simulink model "modeFinalPP"  (R2021b)
settings: Solver=ode23s  StartTime=0.0  StopTime=150  RelTol=1e-3
model workspace (MAT data in the model file):
  firstWarning = 1
  originalScenarioChecksum = '114339432DE22364D47BB28FC96DC10C'
undefined symbols (not defined in the file or in its folder): Acceleration, ActorID, AngularVelocity, curvature, DefaultGear, DEND_B, DEND_S, DEND_T, direction, gradbp, L, ld, LF, LR, MAX_BRAKE, MAX_STEER, MAX_TORQUE, MCAR, MIN_BRAKE, MIN_STEER, MIN_TORQUE, NUMD_B, NUMD_S, NUMD_T, Pitch, point_intersection, PoseRef, Position, psi_o, R, Roll, RRdamp, scenario, sigbuilder_block, STEER_RATIO, stopSign_ID, Tdead, thetaRefs, TL_ID, TrackWidth, Ts, ts, Vdead, Velocity, X_o, xRef2s, Y_o, Yaw, yRef2s
libraries: drivingvehiclecontroller x2, simulink x2, drivingscenarioandsensors x2, simulink_extras x1, autolibshared x1, vehdynlibviscommon x1, vehdynlibsteering x1
(part 2 of 2)

== stateflow chart modeFinalPP/Chart ==
  state Navigation
    state RailCrossing
      state Approaching
        en,du:
        VelCmd = ApproachingSpeed;
      state Stop
        en,du:
        VelCmd = 0;
        % apply brakes directly?
      state ExitScene
        en,du:
        ExitFlag = 1;
      state Transition
        en,du:
        VelCmd = SceneSpeed;
      (default) -> Navigation.RailCrossing.Approaching
      Navigation.RailCrossing.Approaching -> Navigation.RailCrossing.Stop : [D2S <= SDist]
      Navigation.RailCrossing.Stop -> Navigation.RailCrossing.Transition : [after(3,sec)]
      Navigation.RailCrossing.Transition -> Navigation.RailCrossing.ExitScene : [SDir == 'S']
    state RoundAbout
      state Approaching
        en,du:
        VelCmd = ApproachingSpeed;
      state Stop
        en,du:
        VelCmd = 0;
        % apply brakes directly?
      state ExitScene
        en,du:
        ExitFlag = 1;
      state Transition
        en,du:
        VelCmd = SceneSpeed;
      (default) -> Navigation.RoundAbout.Approaching
      Navigation.RoundAbout.Approaching -> Navigation.RoundAbout.Stop : [D2S <= SDist]
      Navigation.RoundAbout.Stop -> Navigation.RoundAbout.Transition : [after(3,sec)]
      Navigation.RoundAbout.Transition -> Navigation.RoundAbout.ExitScene : [SDir == 'S']
    state DestCheck
      en,du:
      % dest reached?
      (default) -> (junction 47)
      (junction 47) -> (junction 48) [order 1] : [D2D < 1]
      (junction 47) -> (junction 49) [order 2] : {DestReached = 0;}
      (junction 48) -> (junction 50) : {DestReached = 1;}
      (junction 50) -> (junction 49)
      (junction 49) -> (junction 51)
    state TrafficLight
      state Approaching
        en,du:
        VelCmd = ApproachingSpeed;
      state Stop
        en,du:
        VelCmd = 0;
        % apply brakes directly?
      state ExitScene
        en,du:
        ExitFlag = 1;
      state Transition
        en,du:
        VelCmd = SceneSpeed;
      (default) -> Navigation.TrafficLight.Approaching
      Navigation.TrafficLight.Approaching -> Navigation.TrafficLight.Stop : [D2S <= SDist]
      Navigation.TrafficLight.Stop -> Navigation.TrafficLight.Transition : [after(3,sec)]
      Navigation.TrafficLight.Transition -> Navigation.TrafficLight.ExitScene : [SDir == 'S']
    state SceneRecognition
      en,du:
      VelCmd = 5;
      ExitFlag = 0;
    state Go
      du:
      VelCmd = 5;
    state StopSign
      state Approaching
        en,du:
        VelCmd = ApproachingSpeed;
      state Stop
        en,du:
        VelCmd = 0;
        % apply brakes directly?
      state ExitScene
        en,du:
        ExitFlag = 1;
      state Transition
        en,du:
        VelCmd = SceneSpeed;
      (default) -> Navigation.StopSign.Approaching
      Navigation.StopSign.Approaching -> Navigation.StopSign.Stop : [D2S <= SDist]
      Navigation.StopSign.Stop -> Navigation.StopSign.Transition : [after(3,sec)]
      Navigation.StopSign.Transition -> Navigation.StopSign.ExitScene : [SDir == 'S']
    SceneRecognition -> RailCrossing [order 1] : [Scene == 4]
    RailCrossing -> Go : [ExitFlag == 1]
    SceneRecognition -> RoundAbout [order 4] : [Scene == 3]
    RoundAbout -> Go : [ExitFlag == 1]
    (default) -> DestCheck
    SceneRecognition -> TrafficLight [order 3] : [Scene == 2]
    DestCheck -> SceneRecognition : [DestReached == 0]
    SceneRecognition -> StopSign [order 2] : [Scene == 1]
    TrafficLight -> Go : [ExitFlag == 1]
    StopSign -> Go : [ExitFlag == 1]
    Go -> DestCheck : [Scene == 0]
  state Stationary
    du:
    VelCmd = 0;
  (default) -> Stationary
  Stationary -> Navigation : [Navigate == 1]
  Navigation -> Stationary : [Navigate == 0 || DestReached == 1]
  data: SDir input; ApproachingSpeed input; SceneSpeed input; SDist input; D2S input; Scene input; VelCmd output; DestReached local; Navigate input; ExitFlag local; D2D input
